simulink model "lin_rocketmodel"  (R2019b)
settings: Solver=VariableStepAuto  StartTime=0.0  StopTime=40  RelTol=1e-9
values from neighbouring files (symbols this model uses):
  A = A*(v_phi(k,i)*s^i)    [Roberts_Q_design.m]    (also in main_fmincon.m = []; rocket_model.m = [0,1,0,0,0,0; ss_model.mat = [0  0; 1  0]; verif.m = [0,1;0,0])
  B = B*(s-alpha(i))    [Roberts_Q_design.m]    (also in controller_design.m = B*C(2); main_yp_fminunc.m = B*C(2); rocket_controllerdesign.m = B*C(2); rocket_controllerdesign_z.m = B*C(2))
  C = [0,1]    [controller_design.m]    (also in main_yp_fminunc.m; rocket_controllerdesign.m; rocket_controllerdesign_z.m; rocket_model.m = eye(6))
  D = 0    [rocket_model.m]    (also in ss_model.mat; verif.m)
  Ts = 0.001    [main_rocketmodel.m]    (also in main_sim_rocket.m; sim_lin.m; square_sig.m; sum_squares_sig.m)
  z_0 = 4000    [main_rocketmodel.m]    (also in main_sim_rocket.m; sim_lin.m; test_bangbang.m)
settings Model: Creator=bia  LastModifiedBy=bia
settings DataIOCC: ExternalInput=[t, thrust, gimbal]  LoadExternalInput=on

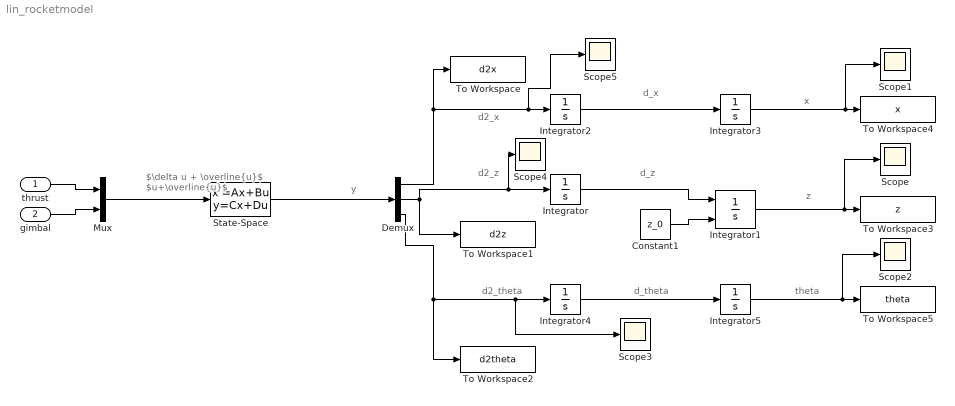
== system lin_rocketmodel ==
  note: d2_theta
  note: d_theta
  note: theta
  note: y
  note: $\delta u + \overline{u}$ $u+\overline{u}$
  note: d2_z
  note: d2_x
  note: d_z
  note: d_x
  note: x
  note: z
  thrust : Inport
  "gimbal " : Inport  Port=2
  Constant1 : Constant  Value=z_0
  Demux : Demux  Outputs=3
  Integrator : Integrator
  Integrator1 : Integrator  InitialConditionSource=external  InitialCondition=4000  LimitOutput=on  LowerSaturationLimit=0
  Integrator2 : Integrator
  Integrator3 : Integrator  LowerSaturationLimit=0
  Integrator4 : Integrator
  Integrator5 : Integrator  LowerSaturationLimit=0
  Mux : Mux  Inputs=2
  Scope{,1..5} (6 alike) : Scope
  State-Space : StateSpace  A=A  B=B  C=C  D=D  InitialCondition=0
  To Workspace : ToWorkspace  VariableName=d2x  SampleTime=Ts
  To Workspace1 : ToWorkspace  VariableName=d2z  SampleTime=Ts
  To Workspace2 : ToWorkspace  VariableName=d2theta  SampleTime=Ts
  To Workspace3 : ToWorkspace  VariableName=z  SampleTime=Ts
  To Workspace4 : ToWorkspace  VariableName=x  SampleTime=Ts
  To Workspace5 : ToWorkspace  VariableName=theta  SampleTime=Ts
  wires:
  thrust/1 -> Mux/1
  State-Space/1 -> Demux/1
  Demux/1 -> Scope5/1, Integrator2/1, To Workspace/1
  Demux/2 -> Scope4/1, Integrator/1, To Workspace1/1
  Demux/3 -> To Workspace2/1, Scope3/1, Integrator4/1
  Integrator/1 -> Integrator1/1
  Integrator1/1 -> Scope/1, To Workspace3/1
  Integrator2/1 -> Integrator3/1
  Integrator3/1 -> Scope1/1, To Workspace4/1
  Integrator4/1 -> Integrator5/1
  Integrator5/1 -> Scope2/1, To Workspace5/1
  Constant1/1 -> Integrator1/2
  Mux/1 -> State-Space/1
  "gimbal "/1 -> Mux/2
